simulink model "Experiment_1_cs"  (R2022b)
settings: Solver=ode5  StartTime=0.0  StopTime=30  FixedStep=1/20  RelTol=1e-3
PreLoadFcn:
  | mbxruntime.callbacks.PreLoadFcn(bdroot);
PostLoadFcn:
  | mbxruntime.callbacks.PostLoadFcn(bdroot);
InitFcn:
  | mbxruntime.callbacks.InitFcn(bdroot);
StartFcn:
  | mbxruntime.callbacks.StartFcn(bdroot);
StopFcn:
  | mbxruntime.callbacks.StopFcn(bdroot);
model workspace (MAT data in the model file):
  mbox_table : object (value not decoded)
  model_closed = 0
  sim_status = 0
undefined symbols (not defined in the file or in its folder): blockPath, DiscIntNeverNeededParam, warningInitialVelocity, x0
libraries: PreScanSimulinkLibrary x32, simulink x23, simulink_extras x10
(part 8 of 8)

== matlab function Experiment_1_cs/Cloud Computing Systerm/Dangerous Check/MATLAB Function2 ==
  settings: updateMethod=DISCRETE
  data: no_signal_zone_x input; ego_y input; lane0_y input; target_y output; lane1_y input; lane2_y input; last_target_y input; obs_x_set_gcs input; obs_y_set_gcs input; obs_v_set_gcs input; obs_heading_set_gcs input; obs_ID_set input; ego_x input; ego_v input; ego_heading input; ego_yawrate input; last_target_v input; target_v output; time input; out_state output; has_signal output; danger_level output; action output; collision_info output Bus: collision_info_bus
function [target_y, target_v, out_state, has_signal, danger_level, action, collision_info] = ...
    fcn(no_signal_zone_x, ego_y, lane0_y, lane1_y, lane2_y, last_target_y, ...
        obs_x_set_gcs, obs_y_set_gcs, obs_v_set_gcs, obs_heading_set_gcs, ...
        obs_ID_set, ego_x, ego_v, ego_heading, ego_yawrate, last_target_v, time)


%% ------------------------------------------------------
% Persistent Variables
%% ------------------------------------------------------
persistent first_run stored_target_y stored_target_v state block_until_time
action = 0;
collision_info.obs_id = int32(-1);
collision_info.time = -1;

if isempty(first_run)
    first_run = true;
    stored_target_y = 0;
    stored_target_v = 0;
    state = 0;
    block_until_time = 0;
end

%% Parameters
dt = 0.05;
recommond_speed = 15;
lane_width = 3.5;
max_acc = 2;
max_de_acc = -2.5;

ego_heading = wrapToPi(-deg2rad(ego_heading - 90));
lane_y_all = [lane0_y, lane1_y, lane2_y];

%% Signal availability
has_signal = (ego_x < no_signal_zone_x);

%% =============== CASE 1: LOST SIGNAL ===================
if ~has_signal
    stored_target_v = 0;
    stored_target_y = 0;
    state = 0;

    danger_level = calc_lost_signal_danger( ...
        ego_x, ego_y, ego_heading, ...
        obs_x_set_gcs, obs_y_set_gcs, obs_v_set_gcs, obs_heading_set_gcs, ...
        obs_ID_set, lane_y_all, lane_width);

    target_v = stored_target_v;
    target_y = stored_target_y;
    out_state = state;
    action = 0;
    return;
end

%% =============== FIRST RUN ===================
if first_run
    [~, idx_lane] = min(abs(ego_y - lane_y_all));
    stored_target_y = lane_y_all(idx_lane);
    stored_target_v = recommond_speed;

    first_run = false;

    target_y = stored_target_y;
    target_v = stored_target_v;
    out_state = state;
    danger_level = 0;
    action = 0;
    return;
end

%% =============== NORMAL MODE ===================
stored_target_y = last_target_y;
stored_target_v = last_target_v;

%% Danger Analysis
[danger, tx_lane] = analyze_danger( ...
    ego_x, ego_y, ego_v, ego_heading, ...
    obs_x_set_gcs, obs_y_set_gcs, obs_v_set_gcs, obs_heading_set_gcs, obs_ID_set, ...
    lane_y_all, lane_width);

% Determine lane index (scalar)
lane_idx = 1;
min_val = abs(stored_target_y - lane_y_all(1));
for ii = 2:3
    if abs(stored_target_y - lane_y_all(ii)) < min_val
        min_val = abs(stored_target_y - lane_y_all(ii));
        lane_idx = ii;
    end
end

is_danger = danger(lane_idx, 1);
t_lane  = tx_lane(lane_idx, 1);
x_lane  = tx_lane(lane_idx, 2);
if is_danger
    collision_info.obs_id = int32(danger(lane_idx, 2));
    collision_info.time = t_lane;
end

%% --------------------- State Machine ---------------------
switch state

case 0   % KEEP
    action = 0;
    block_until_time = time;

    if is_danger
        state = 1;
    else
        stored_target_v = min(stored_target_v + max_acc*dt, recommond_speed);
    end

case 1   % BRAKE
    if is_danger
        d_brake = ego_v^2 / (2*abs(max_de_acc));
        dx_conflict = x_lane - ego_x;

        if d_brake < dx_conflict - 6
            stored_target_v = last_target_v + max_de_acc * dt;
            action = 2;

            obs_id = danger(lane_idx,2);
            idx_obs = find(obs_ID_set == obs_id, 1);
            if isempty(idx_obs), idx_obs = 1; end

            vy = obs_v_set_gcs(idx_obs) * sin(obs_heading_set_gcs(idx_obs));

            block_until_time = time + t_lane + (lane_width/2)/max(abs(vy),0.01) + 0.5;

        else
            % change lane
            
            if lane_idx == 1
                cand = 2;
            elseif lane_idx == 3
                cand = 2;
            else
                cand = [1, 3];
            end
        
            % 从候选车道里找一个安全车道
            new_lane = lane_idx; % 默认保持
            for ci = 1:length(cand)
                if ~danger(cand(ci),1)
                    new_lane = cand(ci);
                    break;
                end
            end

            stored_target_y = lane_y_all(new_lane);
            state = 2;
            action = 3;
        end

        % failsafe: too slow but still dangerous
        if ego_v < 5 && is_danger
            new_lane = lane_idx;
            found = false;

            for li = 1:3
                if danger(li,1)==false
                    new_lane = li;
                    found = true;
                    break;
                end
            end

            if ~found
                action = 4;
            else
                stored_target_y = lane_y_all(new_lane);
                state = 2;
            end
        end

    else
        state = 3;
        action = 1;
    end

case 2   % CHANGE LANE
    block_until_time = time + 0.5;
    stored_target_v = last_target_v;
    state = 3;
    action = 3;

case 3   % BLOCK
    if time >= block_until_time
        state = 0;
    end
    stored_target_v = last_target_v;
    action = 1;

end

%% Outputs
target_y = stored_target_y;
target_v = stored_target_v;
out_state = state;
danger_level = 0;

end  % END fcn


%% =====================================================================
%%                        analyze_danger
%% =====================================================================
function [danger, tx_lane] = analyze_danger( ...
    ego_x, ego_y, ego_v, ego_heading, ...
    obs_x, obs_y, obs_v, obs_h, obs_ID, lane_y, lane_width)

N = length(obs_ID);

danger = zeros(3,2);         % [is_danger, obs_ID]
tx_lane = 99 * ones(3,2);    % [t_lane, x_at_lane]

for i = 1:N
    if isnan(obs_ID(i))
        continue;
    end

    % First-level screening
    risk_flag = ray_intersect(ego_x, ego_y, ego_heading, ...
                              obs_x(i), obs_y(i), obs_h(i));
    if ~risk_flag
        continue;
    end

    vy = obs_v(i) * sin(obs_h(i));
    vx = obs_v(i) * cos(obs_h(i));

    for j = 1:3

        % --------- Compute t_lane ----------
        if abs(obs_y(i) - lane_y(j)) < lane_width/2
            t_lane = 0;

        elseif abs(vy) < 0.01
            t_lane = inf;

        else
            t_lane = (lane_y(j) - obs_y(i)) / vy;
            if t_lane <= 0
                t_lane = inf;
            end
        end

        if isinf(t_lane)
            continue;
        end

        % --------- Compute collision x ------
        x_lane   = obs_x(i) + vx * t_lane;
        ego_x_t  = ego_x + ego_v * t_lane * cos(ego_heading);

        % --------- Risk Conditions ----------
        cond1 = (t_lane < 4);
        cond2 = abs(ego_x_t - x_lane) < max(10, 2 * ego_v);

        if cond1 || cond2
            danger(j,1) = 1;
            danger(j,2) = obs_ID(i);
            tx_lane(j,1) = t_lane;
            tx_lane(j,2) = x_lane;
        end

    end
end

end


%% =====================================================================
%%                     calc_lost_signal_danger
%% =====================================================================
function danger_level = calc_lost_signal_danger(ego_x, ego_y, ego_heading, ...
    obs_x, obs_y, obs_v, obs_h, obs_ID, lane_y_all, lane_width)

danger_level = 0;

N = length(obs_ID);
if N == 0
    return;
end

% Find nearest lane
lane_idx = 1;
min_dist = abs(ego_y - lane_y_all(1));
for j = 2:3
    if abs(ego_y - lane_y_all(j)) < min_dist
        min_dist = abs(ego_y - lane_y_all(j));
        lane_idx = j;
    end
end

t_min = 1e9;  % scalar

for k = 1:N
    if isnan(obs_ID(k))
        continue;
    end

    vy = obs_v(k) * sin(obs_h(k));
    vx = obs_v(k) * cos(obs_h(k));

    % ----- Compute t_lane -----
    if abs(obs_y(k) - lane_y_all(lane_idx)) < lane_width/2
        t_lane = 0;

    elseif abs(vy) < 0.01
        continue;

    else
        t_lane = (lane_y_all(lane_idx) - obs_y(k)) / vy;
        if t_lane <= 0
            continue;
        end
    end

    if t_lane < t_min
        t_min = t_lane;
    end
end

% ----- Level mapping -----
if t_min < 3
    danger_level = 3;
elseif t_min < 5
    danger_level = 2;
elseif t_min < 10
    danger_level = 1;
end

end


%% =====================================================================
%%                       ray_intersect
%% =====================================================================
function is_possible = ray_intersect(x1,y1,h1, x2,y2,h2)

% Unit heading vectors
H1 = [cos(h1), sin(h1)];
H2 = [cos(h2), sin(h2)];

% Relative position
r = [x2 - x1, y2 - y1];

% Heading difference
diff_rad = abs(wrapToPi(h1 - h2));

% Nearly parallel → use min distance
if diff_rad < deg2rad(2)
    dist_min = abs(r(1)*H1(2) - r(2)*H1(1));
    is_possible = (dist_min < 5);
    return;
end

% Cross product (denominator)
den = H1(1)*H2(2) - H1(2)*H2(1);

if abs(den) < 1e-6
    dist_min = abs(r(1)*H1(2) - r(2)*H1(1));
    is_possible = (dist_min < 5);
    return;
end

% Solve ray intersection
t1 = ( r(1)*H2(2) - r(2)*H2(1) ) / den;
t2 = ( r(1)*H1(2) - r(2)*H1(1) ) / den;

if (t1 > 0) && (t2 > 0)
    is_possible = true;
    return;
end

% Intersection behind, but close enough → possible
dist_min = abs(r(1)*H1(2) - r(2)*H1(1));
is_possible = (dist_min < 5);

end

== matlab function Experiment_1_cs/Cloud Computing Systerm/Dangerous Check/平面美化前 ==
  data: has_signal input; action input; danger_level input; obs_x input; obs_y input; obs_v input; obs_heading input; obs_id input; host_x input; host_y input; host_v input; host_heading input; target_y input
function plot_obstacles_gcs(has_signal, action, danger_level, obs_x, obs_y, obs_v, obs_heading, obs_id, host_x, host_y, host_v, host_heading, target_y)
% 绘制 GCS 下的自车与障碍物（固定视野）——适用于 Simulink

coder.extrinsic('figure','clf','hold','grid','axis','xlim','ylim','xlabel','ylabel','title');
coder.extrinsic('plot','quiver','text','fill','legend','sprintf');

status_text = '';
coder.varsize('status_text',[1 200]);   % 最大 200 chars

persistent figCreated;
persistent prev_action;

if isempty(prev_action)
    prev_action = 0;    % 默认上一周期为正常驾驶
end

%% 
% 图初始化
if isempty(figCreated)
    figure(200);
    figCreated = true;
end

figure(200);
clf; hold on; grid on; axis equal;

%% 
% 固定视野范围 
forward_range = 120;
back_range    = 20;
side_range    = 70;

xlim([host_x - back_range, host_x + forward_range]);
ylim([host_y - side_range, host_y + side_range]);

xlabel('X_{GCS} (m)');
ylabel('Y_{GCS} (m)');
title('Obstacle Positions in Global Coordinate System (Local View)');

%% ============================
% 自车矩形（朝向 host_heading）
% ============================
Lh = 5;
Wh = 2;

host_heading_rad = deg2rad(-host_heading + 90);

rect = [
    Lh/2,  Wh/2;
    Lh/2, -Wh/2;
    -Lh/2, -Wh/2;
    -Lh/2,  Wh/2
    ];

R = [cos(host_heading_rad) -sin(host_heading_rad);
    sin(host_heading_rad)  cos(host_heading_rad)];

rect_rot = (R * rect')';
rect_final = rect_rot + [host_x, host_y];

fill(rect_final(:,1), rect_final(:,2), ...
    [0.2 0.6 1.0], 'FaceAlpha',0.4, 'EdgeColor','b', 'LineWidth',2);

text(host_x, host_y - 3.5, 'Host Car', ...
    'Color','b','FontSize',12,'FontWeight','bold');
text(host_x, host_y + 3.5, sprintf('%.1f m/s', host_v), ...
    'Color','b','FontSize',12,'FontWeight','bold');

%% ============================
% 绘制障碍物
% ============================
for i = 1:length(obs_x)
    if isnan(obs_x(i)), continue; end

    ox = obs_x(i);
    oy = obs_y(i);
    v  = obs_v(i);
    hd = obs_heading(i);
    oid = obs_id(i);

    % 速度箭头
    quiver(ox, oy, v*cos(hd), v*sin(hd), 1.5, 'b', 'LineWidth', 1.5);
    text(ox + 5, oy + 3.5, sprintf('%.1f m/s', v), ...
    'Color','b','FontSize',10,'FontWeight','bold');

    % 车辆障碍物
    if oid == 42 || oid == 54 || oid == 38
        L = 5; W = 2;

        rect = [
            L/2,  W/2;
            L/2, -W/2;
            -L/2, -W/2;
            -L/2,  W/2
            ];

        R = [cos(hd) -sin(hd); sin(hd) cos(hd)];
        rect_rot = (R * rect')';
        rect_final = rect_rot + [ox, oy];

        fill(rect_final(:,1), rect_final(:,2), [0.3 0.8 0.3], ...
            'FaceAlpha',0.4, 'EdgeColor','g', 'LineWidth',2);

        txt = sprintf('Car(%d)', int32(oid));
        text(ox, oy - 5, txt, 'Color','g','FontSize',12,'FontWeight','bold');

    else
        % 普通障碍物
        plot(ox, oy, 'ro', 'MarkerFaceColor', 'r');
        text(ox, oy -3.5, sprintf('%d', int32(oid)), ...
            'Color','b','FontSize',12,'FontWeight','bold');
    end
end

if ~isnan(target_y)
    plot([host_x, host_x + forward_range], ...
        [target_y, target_y], ...
        'B--', 'LineWidth', 0.5);

end

% 无信号区域分级提醒
%% ============================
% 显示信号状态 + 危险等级
% ============================

if ~has_signal
    status_text = sprintf('\\color{red}No Signal  Danger Level %d', danger_level);
else
    % 1) 先决定应该显示哪个 action
    show_action = action;

    % action==1 则显示上一周期的动作，不更新 prev_action
    if action == 1
        show_action = prev_action;
    end

    % 2) 根据 show_action 生成语句
    if show_action == 0
        status_text = sprintf('\\color{green}Has Signal  Normal Drive');
    elseif show_action == 2
        status_text = sprintf('\\color{blue}Has Danger, Decelerate');

    elseif show_action == 3
        status_text = sprintf('\\color{magenta}Has Danger, Lane Change');

    else
        % 防御性代码，不可能走到这里
        status_text = sprintf('\\color{green}Has Signal');
    end

    % 3) action==1 时不更新 prev_action，其它情况下更新
    if action ~= 1
        prev_action = action;
    end
end

% 固定显示在视图左上角
if ~isempty(status_text)
    text(host_x - back_range + 2, host_y + side_range - 2, ...
        status_text, ...
        'FontSize', 12, 'FontWeight', 'bold', ...
        'Interpreter','tex');   % 支持颜色文字
end


legend('Velocity','Host');

end

== matlab function Experiment_1_cs/Cloud Computing Systerm/Dangerous Check/平面美化后1 ==
  data: has_signal input; action input; danger_level input; obs_x input; obs_y input; obs_v input; obs_heading input; obs_id input; host_x input; host_y input; host_v input; host_heading input; target_y input; collision_info input
function plot_obstacles_gcs(has_signal, action, danger_level, ...
    obs_x, obs_y, obs_v, obs_heading, obs_id, ...
    host_x, host_y, host_v, host_heading, target_y, collision_info)

coder.extrinsic('figure','clf','hold','grid','axis','xlim','ylim',...
    'xlabel','ylabel','title','plot','quiver','text','fill','legend','sprintf');

%% Persistent for UI
persistent figCreated;
persistent prev_action;

%% Persistent for trajectory memory
persistent traj_ids;        % [1×MAX_OBJ]  保存每个轨迹对应的ID
persistent traj_len;        % [1×MAX_OBJ]  每个轨迹当前长度
persistent traj_history;    % cell: 每个 cell 是 [MAX_POINTS×2] 的数组

MAX_OBJ    = 50;       % 最大障碍物数量
MAX_POINTS = 200;      % 每个障碍物最多保存 200 个点

%% Init persistent trajectory cache
if isempty(traj_ids)
    traj_ids     = zeros(1,MAX_OBJ);          % 0 表示空槽
    traj_len     = zeros(1,MAX_OBJ);          % 每个轨迹当前长度
    traj_history = cell(1,MAX_OBJ);

    % Init trajectory buffers
    for i = 1:MAX_OBJ
        traj_history{i} = zeros(MAX_POINTS,2);   % 每个障碍物的轨迹缓存
    end
end

if isempty(prev_action)
    prev_action = 0;
end

%% Init figure
if isempty(figCreated)
    figure(200);
    figCreated = true;
end

figure(200);
clf; hold on; axis equal;

%% UI colors
set(gcf,'Color',[0.08 0.10 0.12]);
set(gca,'Color',[0.10 0.12 0.14]);
set(gca,'XColor',[0.6 0.7 0.8],'YColor',[0.6 0.7 0.8]);
grid on; set(gca,'GridAlpha',0.15,'GridColor',[0.5 0.6 0.7]);

%% ranges
forward_range = 120;
back_range = 20;
side_range = 70;

xlim([host_x - back_range, host_x + forward_range]);
ylim([host_y - side_range, host_y + side_range]);

xlabel('X (m)','Color',[0.7 0.8 0.9]);
ylabel('Y (m)','Color',[0.7 0.8 0.9]);
title('Local View','Color',[0.8 0.9 1],'FontWeight','bold');

%% Draw Ego
Lh = 5; Wh = 2;
host_heading_rad = deg2rad(-host_heading + 90);

rect = [ Lh/2 Wh/2; Lh/2 -Wh/2; -Lh/2 -Wh/2; -Lh/2 Wh/2 ];
R = [cos(host_heading_rad) -sin(host_heading_rad); sin(host_heading_rad) cos(host_heading_rad)];
rect_rot = (R*rect')'; 
rect_final = rect_rot + [host_x, host_y];

fill(rect_final(:,1)-0.2, rect_final(:,2)-0.2,[0 0 0],'FaceAlpha',0.25,'EdgeColor','none');
fill(rect_final(:,1), rect_final(:,2),[0.15 0.45 0.95],'FaceAlpha',0.55,'EdgeColor',[0.5 0.7 1],'LineWidth',2);
text(host_x-18, host_y, 'Ego','Color',[0.6 0.8 1],'FontSize',12,'FontWeight','bold');
text(host_x-15, host_y+5.5, sprintf('%.1f m/s', host_v),'Color',[0.7 0.9 1],'FontSize',12);

%% Draw Obstacles + Trajectories
for i = 1:length(obs_x)
    if isnan(obs_x(i)), continue; end

    ox = obs_x(i); 
    oy = obs_y(i);
    v  = obs_v(i);
    hd = obs_heading(i);
    oid = obs_id(i);

    %% ============================
    % ⭐ 更新/写入轨迹缓存
    %% ============================
    idx = 0;

    % 查找已有 ID
    for k = 1:MAX_OBJ
        if traj_ids(k) == oid
            idx = k;
            break;
        end
    end

    % 若无 → 找空槽
    if idx == 0
        for k = 1:MAX_OBJ
            if traj_ids(k) == 0
                traj_ids(k) = oid;
                idx = k;
                break;
            end
        end
    end

    if idx == 0
        continue; % 没槽了，跳过
    end

    % 写入轨迹点
    L = traj_len(idx) + 1;
    if L > MAX_POINTS
        L = MAX_POINTS;
    end

    traj_len(idx) = L;
    traj_history{idx}(L,:) = [ox oy];

    %% ============================
    % ⭐ 绘制已有轨迹
    %% ============================
    Ldraw = traj_len(idx);
    traj = traj_history{idx}(1:Ldraw,:);

    plot(traj(:,1), traj(:,2), '-', ...
        'Color',[0.3 0.7 1 0.30], 'LineWidth',1.2);

    %% Vel arrow
    quiver(ox, oy, v*cos(hd), v*sin(hd),1.3,'Color',[0.55 0.75 1],'LineWidth',1.2);
    text(ox+10, oy, sprintf('%.1f m/s', v),'Color',[0.75 0.85 1],'FontSize',10);

    %% ⭐ 碰撞信息
    if ~isempty(collision_info) && ...
       (oid == collision_info.obs_id) && ...
        collision_info.time < 99

        text(ox+25, oy, sprintf('t=%.1f s', collision_info.time), ...
            'Color',[1 0.9 0.3],'FontSize',10,'FontWeight','bold');
    end

    %% Draw obstacle
    if oid==42 || oid==54 || oid==38
        % --- Cars
        Lc=5; Wc=2;
        car_rect=[Lc/2 Wc/2; Lc/2 -Wc/2; -Lc/2 -Wc/2; -Lc/2 Wc/2];
        R=[cos(hd) -sin(hd); sin(hd) cos(hd)];
        rr=(R*car_rect')'+[ox oy];

        fill(rr(:,1)-0.1,rr(:,2)-0.1,[0 0 0],'FaceAlpha',0.28,'EdgeColor','none');
        fill(rr(:,1),rr(:,2),[0.15 0.85 0.75],'FaceAlpha',0.55,'EdgeColor',[0.4 1 0.85],'LineWidth',2);
        text(ox, oy-4.5, sprintf('Car %d', oid),'Color',[0.6 1 0.9],'FontSize',11);

    else
        % --- Pedestrians
        plot(ox, oy, 'o','MarkerSize',2,'MarkerEdgeColor',[1 0.5 0.5], ...
            'MarkerFaceColor',[1 0.2 0.2],'LineWidth',1.5);

        text(ox+2.5, oy, sprintf('%d', oid),'Color',[1 0.6 0.6],'FontSize',11);

        % 距离显示
        dist_to_ego = hypot(ox-host_x, oy-host_y);
        text(ox+2.5, oy-3.5, sprintf('%.1f m', dist_to_ego), ...
            'Color',[1 0.8 0.5],'FontSize',10,'FontWeight','bold');
    end
end

%% Ref line
if ~isnan(target_y) && has_signal
    plot([host_x, host_x+forward_range], ...
         [target_y,target_y], '--','Color',[0.6 0.7 1],'LineWidth',1.2);
end

%% Status bar
if ~has_signal
    s = sprintf('\\color{red}No Signal  Danger Level %d', danger_level);
else
    show_action = action;
    if action==1, show_action = prev_action; end

    switch show_action
        case 0, s='\\color{green}Normal Drive';
        case 2, s='\\color{cyan}Decelerate';
        case 3, s='\\color{magenta}Lane Change';
        otherwise, s='\\color{green}Signal OK';
    end

    if action~=1
        prev_action = action;
    end
end

patch([host_x-back_range host_x+forward_range host_x+forward_range host_x-back_range], ...
      [host_y+side_range host_y+side_range host_y+side_range-6 host_y+side_range-6], ...
      [0.1 0.12 0.15],'FaceAlpha',0.45,'EdgeColor','none');

text(host_x-back_range+2, host_y+side_range-2, s, ...
    'Interpreter','tex','FontSize',13,'FontWeight','bold','Color',[0.9 0.95 1]);

legend('Velocity','Host','TextColor',[0.7 0.8 1]);

end

== matlab function Experiment_1_cs/Cloud Computing Systerm/Dangerous Check/平面美化后2 ==
  data: has_signal input; action input; danger_level input; obs_x input; obs_y input; obs_v input; obs_heading input; obs_id input; host_x input; host_y input; host_v input; host_heading input; target_y input; collision_info input
function plot_obstacles_gcs(has_signal, action, danger_level, ...
    obs_x, obs_y, obs_v, obs_heading, obs_id, ...
    host_x, host_y, host_v, host_heading, target_y, collision_info)

coder.extrinsic('figure','clf','hold','grid','axis','xlim','ylim',...
    'xlabel','ylabel','title','plot','quiver','text','fill','legend','sprintf');

status_text = '';
coder.varsize('status_text',[1 200]);

persistent figCreated;
persistent prev_action;

if isempty(prev_action)
    prev_action = 0;
end

%% 初始化图
if isempty(figCreated)
    figure(200);
    figCreated = true;
end

figure(200);
clf; hold on; axis equal;

%% 🌙 ===== 设置车机 UI 深色背景 =====
set(gcf,'Color',[0.08 0.10 0.12]);  % 深灰 + 蓝调
set(gca,'Color',[0.10 0.12 0.14]);  % 稍亮一点背景
set(gca,'XColor',[0.6 0.7 0.8],'YColor',[0.6 0.7 0.8]);
grid on;
set(gca,'GridAlpha',0.15,'GridColor',[0.5 0.6 0.7]);

%% 视野范围
forward_range = 120;
back_range    = 20;
side_range    = 70;

xlim([host_x - back_range, host_x + forward_range]);
ylim([host_y - side_range, host_y + side_range]);

xlabel('X (m)','Color',[0.7 0.8 0.9]);
ylabel('Y (m)','Color',[0.7 0.8 0.9]);
title('Local View','Color',[0.8 0.9 1],'FontWeight','bold');

%% ============================
% 🚘 自车绘制（矩形 + 阴影）
% ============================
Lh = 5;
Wh = 2;

host_heading_rad = deg2rad(-host_heading + 90);

rect = [
    Lh/2  Wh/2;
    Lh/2 -Wh/2;
    -Lh/2 -Wh/2;
    -Lh/2  Wh/2
    ];

R = [cos(host_heading_rad) -sin(host_heading_rad);
    sin(host_heading_rad)  cos(host_heading_rad)];

rect_rot = (R * rect')';
rect_final = rect_rot + [host_x, host_y];

% 阴影
fill(rect_final(:,1)-0.2, rect_final(:,2)-0.2,...
    [0 0 0],'FaceAlpha',0.25,'EdgeColor','none');

% 主体（蓝色渐变）
fill(rect_final(:,1), rect_final(:,2), ...
    [0.15 0.45 0.95], 'FaceAlpha',0.55, ...
    'EdgeColor',[0.5 0.7 1], 'LineWidth',2);

% 文本
text(host_x - 18, host_y, 'Ego', ...
    'Color',[0.6 0.8 1],'FontSize',12,'FontWeight','bold');

text(host_x - 15, host_y + 5.5, sprintf('%.1f m/s', host_v), ...
    'Color',[0.7 0.9 1],'FontSize',12);


%% ============================
% 🚗 障碍物绘制（车：青色 / 人：红点光晕）
% ============================
for i = 1:length(obs_x)
    if isnan(obs_x(i)), continue; end

    ox = obs_x(i); oy = obs_y(i);
    v  = obs_v(i);
    hd = obs_heading(i);
    oid = obs_id(i);

    % 速度箭头
    quiver(ox, oy, v*cos(hd), v*sin(hd), 1.3, ...
        'Color',[0.55 0.75 1],'LineWidth',1.2);

    text(ox + 10, oy, sprintf('%.1f m/s', v), ...
        'Color',[0.75 0.85 1],'FontSize',10);

    %% === 如果该障碍物是当前危险对象，显示碰撞时间 ===
    if ~isempty(collision_info) ...
            && isfield(collision_info,'obs_id') ...
            && (oid == collision_info.obs_id) ...
            && (collision_info.time < 99)

        text(ox + 30, oy, ...
            sprintf('t=%.1f s', collision_info.time), ...
            'Color',[1 0.9 0.3], ...       % 金黄色
            'FontSize',10, ...
            'FontWeight','bold');
    end


    %% 🚙 车型障碍物（矩形 + 阴影）
    if oid == 42 || oid == 54 || oid == 38
        L = 5; W = 2;

        rect = [
            L/2  W/2;
            L/2 -W/2;
            -L/2 -W/2;
            -L/2  W/2
            ];

        R = [cos(hd) -sin(hd); sin(hd) cos(hd)];
        rr = (R * rect')' + [ox oy];

        % 阴影
        fill(rr(:,1)-0.1, rr(:,2)-0.1, ...
            [0 0 0],'FaceAlpha',0.28,'EdgeColor','none');

        % 主体
        fill(rr(:,1), rr(:,2), ...
            [0.15 0.85 0.75], 'FaceAlpha',0.55, ...
            'EdgeColor',[0.4 1 0.85], 'LineWidth',2);

        text(ox, oy - 4.5, sprintf('Car %d', oid), ...
            'Color',[0.6 1 0.9],'FontSize',11);

    else
        %% 🚶 普通障碍物（红色光晕点）
        plot(ox, oy, 'o', ...
            'MarkerSize',2, ...
            'MarkerEdgeColor',[1 0.5 0.5], ...
            'MarkerFaceColor',[1 0.2 0.2], ...
            'LineWidth',1.5);

        text(ox+2.5, oy, sprintf('%d', oid), ...
            'Color',[1 0.6 0.6],'FontSize',11);
        
        dist_to_ego = hypot(ox - host_x, oy - host_y);
        text(ox + 2.5, oy - 4.0, sprintf('%.1f m', dist_to_ego), ...
            'Color',[1 0.8 0.5], 'FontSize',10, 'FontWeight','bold');
    end
end

%% 参考线
if ~isnan(target_y) && has_signal
    plot([host_x, host_x + forward_range], ...
        [target_y, target_y], ...
        '--','Color',[0.6 0.7 1],'LineWidth',1.2);
end

%% ============================
% 🟦 顶部状态栏（透明背景）
% ============================
if ~has_signal
    status_text = sprintf('\\color{red}No Signal  Danger Level %d', danger_level);
else
    show_action = action;
    if action == 1
        show_action = prev_action;
    end

    switch show_action
        case 0
            status_text = sprintf('\\color{green}Normal Drive');
        case 2
            status_text = sprintf('\\color{cyan}Decelerate');
        case 3
            status_text = sprintf('\\color{magenta}Lane Change');
        otherwise
            status_text = sprintf('\\color{green}Signal OK');
    end

    if action ~= 1
        prev_action = action;
    end
end

% 半透明背景条
patch([host_x-back_range host_x+forward_range host_x+forward_range host_x-back_range], ...
    [host_y+side_range host_y+side_range host_y+side_range-6 host_y+side_range-6], ...
    [0.1 0.12 0.15], 'FaceAlpha',0.45,'EdgeColor','none');

text(host_x - back_range + 2, host_y + side_range - 2, ...
    status_text,'Interpreter','tex', ...
    'FontSize',13,'FontWeight','bold',...
    'Color',[0.9 0.95 1]);

legend('Velocity','Host','TextColor',[0.7 0.8 1]);

end

== matlab function Experiment_1_cs/Cloud Computing Systerm/PathFollower_Preview_1/LateralController/CTRL REFERENCES/Calculate Lateral Error/eml_find_10k_lateral_error_points ==
  data: pvp input size=2; dist_psvehicle output size=10; TrajOffset_x_y_Y input size=3; ActorOffset_Left_Right input; p0 input size=2; PreviewDistance input size=10; Traj_x parameter; Traj_y parameter; Traj_t parameter; Traj_v parameter; RefreshCounter parameter
function dist_psvehicle  = eml_find_10k_lateral_error_points(pvp,TrajOffset_x_y_Y,ActorOffset_Left_Right,p0,PreviewDistance,Traj_x,Traj_y,Traj_t,Traj_v,RefreshCounter)

dist_psvehicle = emlfcn_find_10k_lateral_error_points(pvp,TrajOffset_x_y_Y,ActorOffset_Left_Right,p0,PreviewDistance,Traj_x,Traj_y,Traj_t,Traj_v,RefreshCounter);

% end function

== matlab function Experiment_1_cs/Cloud Computing Systerm/Lat_Control/Simple_lateral_controller/MATLAB Function ==
  data: target_X input; target_Y input; target_Yaw input; steering_wheel_angle_deg output; Ego_X input; Ego_Y input; Ego_Yaw input; Ego_Vx input; steering_ratio input; prev_steer_deg input; dt input
function steering_wheel_angle_deg = StanleyControllerImproved(target_X, target_Y, target_Yaw, ...
    Ego_X, Ego_Y, Ego_Yaw, Ego_Vx, steering_ratio, prev_steer_deg, dt)

% 单位转换
Ego_Vx = Ego_Vx;  % m/s
Ego_Yaw = wrapToPi(deg2rad(-Ego_Yaw + 90));
ref_yaw = wrapToPi(deg2rad(-target_Yaw + 90));


% 横向误差 & 航向误差 

dx = target_X - Ego_X;
dy = target_Y - Ego_Y;
d_yaw = ref_yaw - Ego_Yaw;

d = sqrt(dx^2 + dy^2);

% 横向误差（垂直 ref_yaw 方向）
e_lat = -sin(d_yaw) * dx + cos(d_yaw) * dy;

% 航向误差（保持在 [-pi, pi]）
e_psi = atan2(sin(ref_yaw - Ego_Yaw), cos(ref_yaw - Ego_Yaw));


% Stanley 控制器部分 

k_stanley = 1.8;
a = atan2(k_stanley * e_lat, Ego_Vx + 3);
delta_stanley = e_psi + a;

%  PID 控制器部分 
persistent integral_e_lat prev_e_lat
if isempty(integral_e_lat)
    integral_e_lat = 0;
    prev_e_lat = 0;
end

% PID 参数
Kp = 0.2;
Ki = 0.05;
Kd = 0.001;

% PID 控制器输出
integral_e_lat = integral_e_lat + e_lat * dt;
diff_e_lat = (e_lat - prev_e_lat) / dt;
delta_pid = Kp * e_lat + Ki * integral_e_lat + Kd * diff_e_lat;
prev_e_lat = e_lat;

% 合成最终控制角度 
delta = delta_stanley;

% 限制最大轮角
max_steer = deg2rad(35);
delta = max(-max_steer, min(delta, max_steer));

% 输出方向盘角度 
steering_wheel_angle_deg = rad2deg(delta * steering_ratio);


%==============================
% === Rate Limiter ===
%==============================
% rate_limit = 500; % deg/s
% max_delta = rate_limit * dt;
% steering_wheel_angle_deg = max(prev_steer_deg - max_delta, ...
%                                min(prev_steer_deg + max_delta, steering_wheel_angle_deg));
end

== matlab function Experiment_1_cs/Cloud Computing Systerm/PathFollower_Preview_1/LateralController/CTRL REFERENCES/Find Reference Point (pref0) on Trajectory closest to P0 Point (p0)/eml_find_closest_trajectory_points0 ==
  data: pvp input size=2; Actor_traj_distance output; TrajOffset_x_y_Y input size=3; ActorOffset_Left_Right input; p0 input size=3; Traj_x parameter; Traj_y parameter; Actor_traj_angle output; RefreshCounter parameter
function [Actor_traj_distance,Actor_traj_angle]  = eml_find_closest_trajectory_points0(pvp,TrajOffset_x_y_Y,ActorOffset_Left_Right,p0,Traj_x,Traj_y,RefreshCounter)

[Actor_traj_distance,Actor_traj_angle]  = emlfcn_find_closest_trajectory_points0(pvp,TrajOffset_x_y_Y,ActorOffset_Left_Right,p0,Traj_x,Traj_y,RefreshCounter);

% end function

== matlab function Experiment_1_cs/Audi_A8_Sedan_1/perception module/MATLAB Function1 ==
  data: host_x input; obs_x_set_vcs output; host_y input; host_heading_xy input; obs_range input; obs_theta input; obs_velocity input; obs_velocity_heading input; obs_ID input; obs_y_set_vcs output; obs_velocity_set_vcs output; obs_heading_set_vcs output; obs_ID_set output
function [obs_x_set_vcs, obs_y_set_vcs, obs_velocity_set_vcs, obs_heading_set_vcs, obs_ID_set] = ...
    fcn(host_x, host_y, host_heading_xy, obs_range, obs_theta, obs_velocity, obs_velocity_heading, obs_ID)
% 障碍物 VCS 输出 + 遮挡过滤

% =====================
% 初始化输出（固定 10×1）
% =====================
obs_x_set_vcs       = nan(10,1);
obs_y_set_vcs       = nan(10,1);
obs_velocity_set_vcs = nan(10,1);
obs_heading_set_vcs = nan(10,1);
obs_ID_set          = nan(10,1);

% =====================
% 输入角度转换
% =====================
theta_transfer = -obs_theta * pi / 180;
heading_transfer = (-obs_velocity_heading + host_heading_xy * ones(10,1)) * pi/180;

% =====================
% 坐标变换（传感器系 → VCS）
% =====================
x_transfer = obs_range .* cos(theta_transfer);
y_transfer = obs_range .* sin(theta_transfer);

% =====================
% 填入 VCS（包含无效点）
% =====================
for i = 1:length(obs_range)
    if obs_range(i) ~= 0
        obs_x_set_vcs(i)       = x_transfer(i);
        obs_y_set_vcs(i)       = y_transfer(i);
        obs_heading_set_vcs(i) = heading_transfer(i);
        obs_velocity_set_vcs(i)= obs_velocity(i);
        obs_ID_set(i)          = obs_ID(i);
    end
end

% =====================
% ===== 遮挡过滤 =====
% =====================

% 1) 有效点过滤
valid = ~isnan(obs_x_set_vcs);
ox = obs_x_set_vcs(valid);
oy = obs_y_set_vcs(valid);
ov = obs_velocity_set_vcs(valid);
oh = obs_heading_set_vcs(valid);
oid = obs_ID_set(valid);

if isempty(ox)
    return; % 没有障碍物
end

% 2) 计算角度 + 距离
theta = atan2(oy, ox);           % 朝向角 (-pi~pi)
dist  = sqrt(ox.^2 + oy.^2);     % 距离

% 3) 按角度排序（相邻角度判断遮挡）
[theta_sorted, idx] = sort(theta);
ox = ox(idx);
oy = oy(idx);
ov = ov(idx);
oh = oh(idx);
oid = oid(idx);
dist = dist(idx);

% 4) 遮挡过滤（核心）
angle_threshold = deg2rad(5);
coder.extrinsic('disp');
coder.extrinsic('sprintf');

keep = true(size(ox));
for i = 1:length(ox)
    for j = i+1:length(ox)

        if abs(theta_sorted(j) - theta_sorted(i)) > angle_threshold
            break;
        end

        if dist(j) > dist(i)
            keep(j) = false;
            msg = sprintf('Obs %d blocks out Obs %d', oid(i), oid(j));
            disp(msg);
        else
            keep(i) = false;
            msg = sprintf('Obs %d blocks out Obs %d', oid(j), oid(i));
            disp(msg);
        end
    end
end

% 删除被遮挡的障碍物 ★★★★★
ox  = ox(keep);
oy  = oy(keep);
ov  = ov(keep);
oh  = oh(keep);
oid = oid(keep);

% 最终数量
N = length(ox);

% 清空全部槽位
obs_x_set_vcs(:) = nan;
obs_y_set_vcs(:) = nan;
obs_velocity_set_vcs(:) = nan;
obs_heading_set_vcs(:) = nan;
obs_ID_set(:) = nan;

% 回写输出
obs_x_set_vcs(1:N)        = ox;
obs_y_set_vcs(1:N)        = oy;
obs_velocity_set_vcs(1:N) = ov;
obs_heading_set_vcs(1:N)  = oh;
obs_ID_set(1:N)           = oid;

== matlab function Experiment_1_cs/Cloud Computing Systerm/PathFollower_Preview_1/LateralController/Calculate delta steering error/eml_delta_steering_error ==
  data: v_x_vehicle input; v_x_vehicle_Min input; t_Preview_LatCtrl input; delta_steeringwheeltotal output; v_y_vehicle input; yawrate_vehicle input; CorneringStiffness_Tyres_Front input; CorneringStiffness_Tyres_Rear input; m_vehicle_total input; inertia_z_vehicle_total input; e_Lat input size=10; Pos_x_CoG_Vehicle input; wheelbase input; RefreshCounter parameter
function delta_steeringwheeltotal = eml_delta_steering_error(v_x_vehicle,v_x_vehicle_Min,t_Preview_LatCtrl,v_y_vehicle,yawrate_vehicle,CorneringStiffness_Tyres_Front,CorneringStiffness_Tyres_Rear,m_vehicle_total,inertia_z_vehicle_total,e_Lat,Pos_x_CoG_Vehicle,wheelbase,RefreshCounter)

delta_steeringwheeltotal = emlfcn_delta_steering_error(v_x_vehicle,v_x_vehicle_Min,t_Preview_LatCtrl,v_y_vehicle,yawrate_vehicle,CorneringStiffness_Tyres_Front,CorneringStiffness_Tyres_Rear,m_vehicle_total,inertia_z_vehicle_total,e_Lat,Pos_x_CoG_Vehicle,wheelbase,RefreshCounter);

% end function
